simulink model "flipper"  (R2017b)
settings: Solver=ode4  StartTime=0.0  StopTime=1000  RelTol=1e-3
libraries: vrlib x2
settings Model: Creator=squirrel  LastModifiedBy=squirrel
settings SolverCC: ZeroCrossAlgorithm=Adaptive
settings DebuggingCC: MaxConsecutiveZCsMsg=none

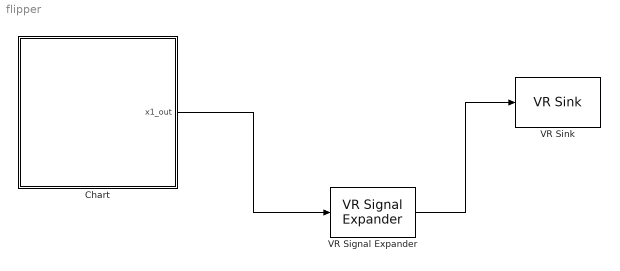
== system flipper ==
  Chart : Stateflow chart  TreatAsAtomicUnit=on
  VR Signal Expander : vrlib/VR Signal Expander  outwidth=3  outidx=[1 2]
      settings: SourceProductName=Simulink 3D Animation  SourceProductBaseCode=VR
  VR Sink : vrlib/VR Sink  InstantiateOnLoad=on  SampleTime=0.05  ViewEnable=on  RemoteChange=off  RemoteView=off  FieldsWritten=Ball.translation.3.1.1.double  WorldFileName=Table.wrl  AutoView=off  VideoDimensions=[]  AllowVariableSize=off
      settings: SourceProductBaseCode=VR
  wires:
  Chart/1(x1_out) -> VR Signal Expander/1
  VR Signal Expander/1 -> VR Sink/1

== stateflow chart flipper/Chart ==
  settings: updateMethod=CONTINUOUS
  state Flipper
    du:
    v1_dot = acc();
    x1_dot = v1;
    %output
    x1_out = x1;
  Flipper -> Flipper [order 2] : [hnd_kontakt == 1]{hnd_refl()}
  (default) -> Flipper : {init()}
  Flipper -> Flipper [order 1] : [wand1_kontakt == 1]{wand1_refl()}
  Flipper -> Flipper [order 3] : [wand3_kontakt == 1]{wand3_refl()}
  Flipper -> Flipper [order 4] : [wand2_kontakt == 1]{wand2_refl()}
  data: a function_output; kontakt1 function_output; kontakt2 function_output; kontakt3 function_output; kontakt_hnd function_output; R constant double =0.25; RHnd constant double =0.8; Hnd local double size=2,1; n1 local double size=2,1; n2 local double size=2,1; n3 local double size=2,1; p1 local double size=2,1; p2 local double size=2,1; p3 local double size=2,1; p4 local double size=2,1; t1 local double size=2,1; t2 local double size=2,1; t3 local double size=2,1; v1 local double size=2,1; x1 local double size=2,1; x1_out output double size=2,1; data local
  data v1 settings: updateMethod=SF_CONTINUOUS_TIME_DATA
  data x1 settings: updateMethod=SF_CONTINUOUS_TIME_DATA
  function a = acc:
    | function a = acc
    |  
    | a = 1 * -n2; % Beschleunigung der Kugel nach unten [m/s^2]
  function init:
    | function init
    |  
    | p1 = [0; 5]; % Position Wand 1
    | p2 = [5; 0]; % Position Wand 1 und 2
    | p3 = [9; 0]; % Position Wand 2 und 3
    | p4 = [10; 7]; % Position Wand 4
    | 
    | Hnd = [6; 2.5]; % Position Hinderniss
    | x1 = [4; 5]; % Startposition Kugel
    | v1 = [0; 0]; % Startgeschwindigkeit Kugel
    | v_dot = 1; % Startbeschleunigung [m/s^2]
    | 
    | t1 = (p2 - p1) / norm(p2 - p1); % Tangentialvektor Wand 1
    | t2 = [1; 0]; % Tangentialvektor Wand 2
    | t3 = (p4 - p3) / norm(p4 - p3); % Tangentialvektor Wand 3
    | 
    | n1 = [-t1(2); t1(1)]; % Normalenvektor Wand 1
    | n2 = [0; 1]; % Normalenvektor Wand 2
    | n3 = [-t3(2); t3(1)]; % Normalenvektor Wand 3
  function wand1_refl:
    | function wand1_refl
    |  
    | vt = v1' * t1; % Geschwindigkeit in tangentiale Richtung zur Wand 1 [m/s]
    | vn = v1' * n1; % Geschwindigkeit in normalen Richtung zur Wand 1 [m/s]
    | v1 = (vt * t1) - (vn * n1); % Geschwindigkeitsvektor zur Wand 1[m/s]
  function kontakt1 = wand1_kontakt:
    | function kontakt1 = wand1_kontakt
    |  
    | d = (x1 - p1)' * n1; % Abstand der Kugel zur Wand 1
    | % Kontakt der Kugel zur Wand 1?
    | if (d <= R)
    |     kontakt1 = 1;
    | else
    |     kontakt1 = 0;
    | end
  function wand2_refl:
    | function wand2_refl
    |  
    | vt = v1' * t2; % Geschwindigkeit in tangentiale Richtung zur Wand 2 [m/s]
    | vn = v1' * n2; % Geschwindigkeit in normalen Richtung zur Wand 2 [m/s]
    | v1 = (vt * t2) - (vn * n2); % Geschwindigkeitsvektor zur Wand 2 [m/s]
  function kontakt2 = wand2_kontakt:
    | function kontakt2 = wand2_kontakt
    |  
    | d = (x1 - p2)' * n2; % Abstand der Kugel zur Wand 2
    | % Kontakt der Kugel zur Wand 2?
    | if (d <= R)
    |     kontakt2 = 1;
    | else
    |     kontakt2 = 0;
    | end
  function wand3_refl:
    | function wand3_refl
    |  
    | vt = v1' * t3; % Geschwindigkeit in tangentiale Richtung zur Wand 3 [m/s]
    | vn = v1' * n3; % Geschwindigkeit in normalen Richtung zur Wand 3 [m/s]
    | v1 = (vt * t3) - (vn * n3); % Geschwindigkeitsvektor zur Wand 3 [m/s]
  function kontakt3 = wand3_kontakt:
    | function kontakt3 = wand3_kontakt
    |  
    | d = (x1 - p3)' * n3; % Abstand der Kugel zur Wand 3
    | % Kontakt der Kugel zur Wand 3?
    | if (d <= R)
    |     kontakt3 = 1;
    | else
    |     kontakt3 = 0;
    | end
  function kontakt_hnd = hnd_kontakt:
    | function kontakt_hnd = hnd_kontakt
    | d = norm(x1 - Hnd); % Abstand der Kugel zum Hinderniss
    | % Kontakt der Kugel zum Hindernis?
    | if (d <= (R + RHnd))
    |     kontakt_hnd = 1;
    | else
    |     kontakt_hnd = 0;
    | end
  function hnd_refl:
    | function hnd_refl
    |  
    | 
    | n = (Hnd - x1) / norm(Hnd - x1); % Normalenvektor Hindernis
    | t = [-n(2); n(1)]; % Tangentialvektor Hindernis
    | 
    | vt = v1' * t; % Geschwindigkeit in tangentiale Richtung zum Hindernis [m/s]
    | vn = v1' * n; % Geschwindigkeit in normalen Richtung zum Hindernis [m/s]
    | v1 = (vt * t) - (vn * n); % Geschwindigkeitsvektor zum Hindernis [m/s]
